simulink model "freewillysimulink"  (R2019b)
settings: Solver=VariableStepAuto  StartTime=0.0  StopTime=100  RelTol=1e-3
PostLoadFcn:
  | m = 10;
  | c = 20;
  | l = 0.25;
  | I = 1;
  | cx = c;
  | cy = c;
  | cth = c;
  | dat = readtable("path.csv");
settings Model: Creator=rbenefo  LastModifiedBy=rbenefo

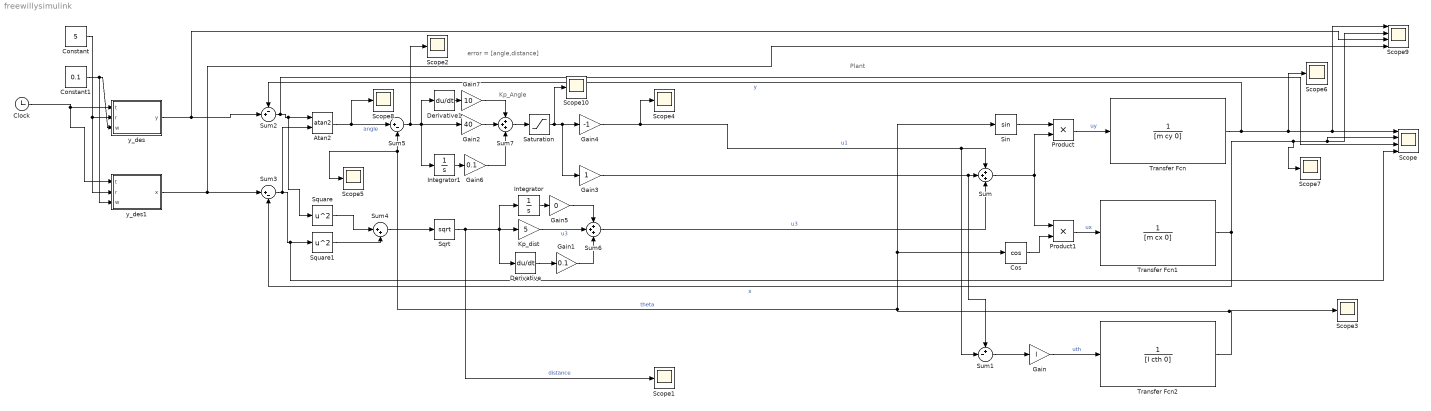
== system freewillysimulink ==
  note: error = [angle,distance]
  note: Kp_Angle
  note: Plant
  Atan2 : Trigonometry  Operator=atan2
  Clock : Clock
  Constant : Constant  Value=5
  Constant1 : Constant  Value=0.1
  Cos : Trigonometry  Operator=cos
  Derivative : Derivative
  Derivative1 : Derivative
  Gain : Gain  Gain=l
  Gain1 : Gain  Gain=0.1
  Gain2 : Gain  Gain=40
  Gain3 : Gain
  Gain4 : Gain  Gain=-1
  Gain5 : Gain  Gain=0
  Gain6 : Gain  Gain=0.1
  Gain7 : Gain  Gain=10
  Integrator : Integrator
  Integrator1 : Integrator
  Kp_dist : Gain  Gain=5
  Product : Product
  Product1 : Product
  Saturation : Saturate  UpperLimit=40  LowerLimit=-40
  Scope : Scope  NumInputPorts=4
  Scope{1..8,10} (9 alike) : Scope
  Scope9 : Scope  NumInputPorts=4
  Sin : Trigonometry
  Sqrt : Sqrt  SaturateOnIntegerOverflow=on
  Square : Math  Operator=square  SignedPower=off  SaturateOnIntegerOverflow=on
  Square1 : Math  Operator=square  SignedPower=off  SaturateOnIntegerOverflow=on
  Sum : Sum  Inputs=+++
  Sum1 : Sum  Inputs=+-|
  Sum2 : Sum  Inputs=-+|
  Sum3 : Sum  Inputs=|+-
  Sum4 : Sum  Inputs=|++
  Sum5 : Sum  Inputs=|+-
  Sum6 : Sum  Inputs=+++
  Sum7 : Sum  Inputs=+++
  Transfer Fcn : TransferFcn  Numerator=1  Denominator=[m cy 0]
  Transfer Fcn1 : TransferFcn  Numerator=1  Denominator=[m cx 0]
  Transfer Fcn2 : TransferFcn  Numerator=1  Denominator=[I cth 0]
  y_des : MATLAB Function  TreatAsAtomicUnit=on
  y_des1 : MATLAB Function  TreatAsAtomicUnit=on
  wires:
  Product/1 -> Transfer Fcn/1  "uy"
  Product1/1 -> Transfer Fcn1/1  "ux"
  Transfer Fcn1/1 -> Scope7/1, Scope9/2, Scope/2, Sum3/2  "x"
  Transfer Fcn2/1 -> Scope3/1, Scope5/1, Sum5/2, Sin/1, Cos/1  "theta"
  Gain/1 -> Transfer Fcn2/1  "uth"
  Gain4/1 -> Scope4/1, Sum1/2, Sum/1  "u1"
  Cos/1 -> Product1/2
  Sin/1 -> Product/1
  Gain3/1 -> Sum1/1, Sum/2
  Sum/1 -> Product1/1, Product/2
  Sum1/1 -> Gain/1
  Transfer Fcn/1 -> Scope6/1, Scope9/1, Scope/1, Sum2/1  "y"
  Sum3/1 -> Atan2/2, Scope/4, Square1/1
  Square/1 -> Sum4/1
  Square1/1 -> Sum4/2
  Sum4/1 -> Sqrt/1
  Sqrt/1 -> Scope1/1, Integrator/1, Derivative/1, Kp_dist/1  "distance"
  Atan2/1 -> Sum5/1, Scope8/1  "angle"
  Sum5/1 -> Derivative1/1, Integrator1/1, Gain2/1, Scope2/1
  Sum6/1 -> Sum/3  "u3"
  Derivative/1 -> Gain1/1
  Kp_dist/1 -> Sum6/2  "u3"
  Gain1/1 -> Sum6/3
  Integrator/1 -> Gain5/1
  Gain5/1 -> Sum6/1
  y_des/1(y) -> Sum2/2, Scope9/3
  Sum2/1 -> Scope/3, Atan2/1, Square/1
  Saturation/1 -> Scope10/1, Gain4/1, Gain3/1
  Sum7/1 -> Saturation/1
  Integrator1/1 -> Gain6/1
  Gain2/1 -> Sum7/2
  Gain6/1 -> Sum7/3
  Derivative1/1 -> Gain7/1
  Gain7/1 -> Sum7/1
  y_des1/1(x) -> Scope9/4, Sum3/1
  Clock/1 -> y_des/1(t), y_des1/1(t)
  Constant/1 -> y_des/2(r), y_des1/2(r)
  Constant1/1 -> y_des1/3(w), y_des/3(w)

== matlab function freewillysimulink/y_des1 ==
  data: t input; x output; r input; w input
function x = fcn(t, r,w)

x = r*sin(w*t);

== matlab function freewillysimulink/y_des ==
  data: t input; y output; r input; w input
function y = fcn(t, r,w)
y = r*cos(w*t)-r;
